simulink model "cstr_open"  (R2021a)
settings: Solver=VariableStepAuto  StartTime=0.0  StopTime=10.0  RelTol=1e-3
settings Model: Creator=User  LastModifiedBy=USER
settings SolverCC: AlgebraicLoopSolver=TrustRegion
settings DebuggingCC: SFMachineParentedDataDiag=warning
settings SFSimCC: CustomCodeUndefinedFunction=UseInterfaceOnly

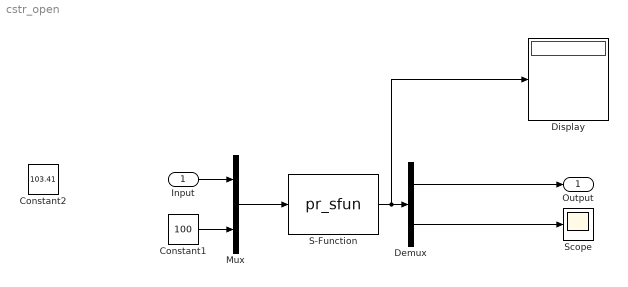
== system cstr_open ==
  Input : Inport
  Constant1 : Constant  Value=100
  Constant2 : Constant  Value=103.41
  Demux : Demux  Outputs=2
  Display : Display
  Mux : Mux  Inputs=2
  S-Function : S-Function  FunctionName=pr_sfun  SFunctionDeploymentMode=off  EnableBusSupport=off
  Scope : Scope
  Output : Outport  VectorParamsAs1DForOutWhenUnconnected=off
  wires:
  Demux/1 -> Output/1
  Mux/1 -> S-Function/1
  S-Function/1 -> Display/1, Demux/1
  Demux/2 -> Scope/1
  Constant1/1 -> Mux/2
  Input/1 -> Mux/1
